simulink model "batterydischargev2"  (R2023b)
settings: Solver=FixedStepAuto  StartTime=0.0  StopTime=15E3  FixedStep=0.2  RelTol=1e-3
values from neighbouring files (symbols this model uses):
  C = 100    [example_thermal_calc.m]
undefined symbols (not defined in the file or in its folder): R2, SoC_t0
libraries: cstextras x2, simulink x1
settings Model: Creator=lricc  LastModifiedBy=lricc
settings OptimizationCC: ReuseModelBlockBuffer=off

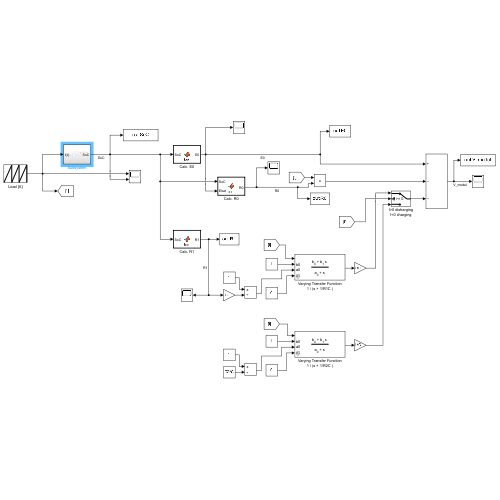
[thumbnail: Simulink's stored preview of the top-level diagram]
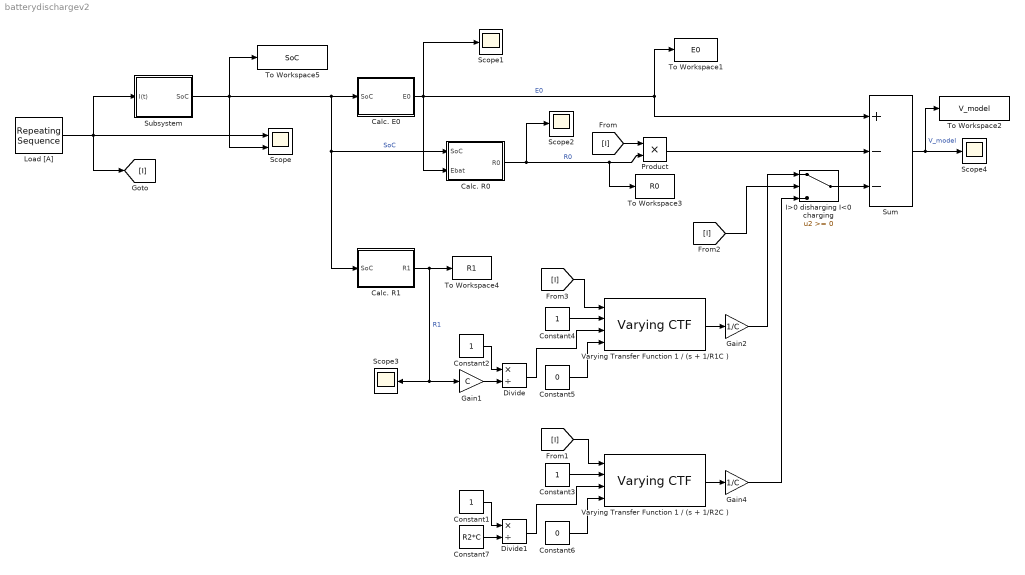
== system batterydischargev2 ==
  Calc. E0 : MATLAB Function  TreatAsAtomicUnit=on
  Calc. R0 : MATLAB Function  TreatAsAtomicUnit=on
  Calc. R1 : MATLAB Function  TreatAsAtomicUnit=on
  Constant{1..4} (4 alike) : Constant
  Constant5 : Constant  Value=0
  Constant6 : Constant  Value=0
  Constant7 : Constant  Value=R2*C
  Divide : Product  Inputs=*/
  Divide1 : Product  Inputs=*/
  Gain1 : Gain  Gain=C
  Gain2 : Gain  Gain=1/C
  Gain4 : Gain  Gain=1/C
  I>0 disharging I<0 charging : Switch  SaturateOnIntegerOverflow=off  InputSameDT=off
  Load [A] : simulink/Sources/Repeating Sequence  rep_seq_t=timeI  rep_seq_y=I
  Product : Product
  Scope : Scope  NumInputPorts=2
  Scope{1..4} (4 alike) : Scope
  Subsystem : Subsystem
  Sum : Sum  Inputs=+--
  To Workspace1 : ToWorkspace  VariableName=E0  SaveFormat=Timeseries  SampleTime=-1
  To Workspace2 : ToWorkspace  VariableName=V_model  SaveFormat=Timeseries  SampleTime=-1
  To Workspace3 : ToWorkspace  VariableName=R0  SaveFormat=Timeseries  SampleTime=-1
  To Workspace4 : ToWorkspace  VariableName=R1  SaveFormat=Timeseries  SampleTime=-1
  To Workspace5 : ToWorkspace  VariableName=SoC  SaveFormat=Timeseries  SampleTime=-1
  Varying Transfer Function 1 / (s + 1/R1C ) : cstextras/Varying CTF  N=1
  Varying Transfer Function 1 / (s + 1/R2C ) : cstextras/Varying CTF  N=1
  wires:
  Load [A]/1 -> [I], Subsystem/1(I(t)), Scope/1
  Subsystem/1(SoC) -> To Workspace5/1, Calc. R1/1(SoC), Calc. R0/1(SoC), Calc. E0/1(SoC), Scope/2  "SoC"
  Calc. E0/1(E0) -> To Workspace1/1, Sum/1, Calc. R0/2(Ebat), Scope1/1  "E0"
  Calc. R0/1(R0) -> To Workspace3/1, Product/2, Scope2/1  "R0"
  Calc. R1/1(R1) -> To Workspace4/1, Gain1/1, Scope3/1  "R1"
  [I] -> Product/1
  Product/1 -> Sum/2
  Sum/1 -> To Workspace2/1, Scope4/1  "V_model"
  Constant4/1 -> Varying Transfer Function 1 / (s + 1/R1C )/2
  Constant5/1 -> Varying Transfer Function 1 / (s + 1/R1C )/4
  [I] -> Varying Transfer Function 1 / (s + 1/R1C )/1
  Divide/1 -> Varying Transfer Function 1 / (s + 1/R1C )/3
  Varying Transfer Function 1 / (s + 1/R1C )/1 -> Gain2/1
  Gain1/1 -> Divide/2
  Constant2/1 -> Divide/1
  Gain2/1 -> I>0 disharging I<0 charging/1
  I>0 disharging I<0 charging/1 -> Sum/3
  Gain4/1 -> I>0 disharging I<0 charging/3
  Constant7/1 -> Divide1/2
  Varying Transfer Function 1 / (s + 1/R2C )/1 -> Gain4/1
  Constant6/1 -> Varying Transfer Function 1 / (s + 1/R2C )/4
  Divide1/1 -> Varying Transfer Function 1 / (s + 1/R2C )/3
  Constant1/1 -> Divide1/1
  [I] -> Varying Transfer Function 1 / (s + 1/R2C )/1
  Constant3/1 -> Varying Transfer Function 1 / (s + 1/R2C )/2
  [I] -> I>0 disharging I<0 charging/2

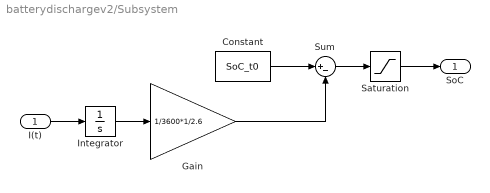
== system batterydischargev2/Subsystem ==
  I(t) : Inport
  Constant : Constant  Value=SoC_t0
  Gain : Gain  Gain=1/3600*1/2.6
  Integrator : Integrator
  Saturation : Saturate  UpperLimit=1  LowerLimit=0
  Sum : Sum  Inputs=|+-
  SoC : Outport
  wires:
  I(t)/1 -> Integrator/1
  Integrator/1 -> Gain/1
  Gain/1 -> Sum/2
  Sum/1 -> Saturation/1
  Constant/1 -> Sum/1
  Saturation/1 -> SoC/1

== matlab function batterydischargev2/Calc. E0 ==
  data: SoC input; E0 output
function E0 = fcn(SoC)
ebat0 = 3.288;
ebat1 = 1.813;
ebat2 = -4.205;
ebat3 = 5.306;
ebat4 = -2.03;

E0 = ebat0 + ebat1.*SoC + ebat2.*SoC^2 + ebat3.*SoC^3 + ebat4.*SoC^4;

== matlab function batterydischargev2/Calc. R1 ==
  data: SoC input; R1 output
function R1 = fcn(SoC)
dint0 = 0.065;
dint1 = -0.057;
dint2 = -0.029;
dint3 = 0.161;
dint4 = -0.116;

R1 = dint0 + dint1.*SoC + dint2.*SoC^2 + dint3.*SoC^3 + dint4.*SoC^4;

== matlab function batterydischargev2/Calc. R0 ==
  data: SoC input; R0 output; Ebat input
function R0 = fcn(SoC,Ebat)
rsint0 = 0.053;
rsint1 = 0.005;
rsint2 = 0.004;
rsint3 = -2;
rsint4 = 3.6;

R0 = rsint0 + rsint1*Ebat + rsint2*exp(rsint3*(Ebat-rsint4));
